simulink subsystem "rate_controller"  (R2021a)
settings: Solver=VariableStepAuto  StartTime=0.0  StopTime=10.0  RelTol=1e-3
undefined symbols (not defined in the file or in its folder): C_rate, DiscIntNeverNeededParam
settings Model: Creator=EpEp  LastModifiedBy=EpEp

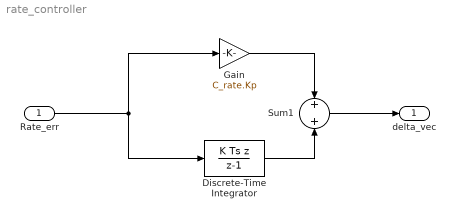
== system rate_controller ==
  Rate_err : Inport
  Discrete-Time Integrator : DiscreteIntegrator  IntegratorMethod=Integration: Backward Euler  gainval=C_rate.Ki  SampleTime=C_rate.Ts  LimitOutput=on  UpperSaturationLimit=10  LowerSaturationLimit=-10  ICPrevOutput=DiscIntNeverNeededParam  ICPrevScaledInput=DiscIntNeverNeededParam
  Gain : Gain  Gain=C_rate.Kp
  Sum1 : Sum  Inputs=+|+
  delta_vec : Outport
  wires:
  Rate_err/1 -> Discrete-Time Integrator/1, Gain/1
  Discrete-Time Integrator/1 -> Sum1/2
  Gain/1 -> Sum1/1
  Sum1/1 -> delta_vec/1
